simulink model "SMC_simulink_model"  (R2022a)
settings: Solver=VariableStepAuto  StartTime=0.0  StopTime=25  MaxStep=1e-3  RelTol=1e-3
InitFcn:
  | clear
  | clc
  | %% dati
  | w0 = 5.278;
  | alfa1 = w0^2;
  | alfa3 = -1.402*w0^2;
  | alfa5 = 0.271*w0^2;
  | mu1 = 0.086;
  | mu3 = 0.1080;
  | %% parametri SMC
  | mu = 1;
  | P = [1 3]';
  | x0 = [-1.2 -0.18]';
  | xd = [0 0]';
  | %disturbi e variazione parametrica
  | Ad = 0; %ampiezza disturbo
  | fd = 2; %fequenza disturbo
  | epsilon = 0.01; %boundary layer
  | alfa1_hat = 0.8*w0^2
settings Model: Creator=user  LastModifiedBy=user
settings SolverCC: ZeroCrossAlgorithm=Adaptive
settings DebuggingCC: IgnoredZcDiagnostic=none

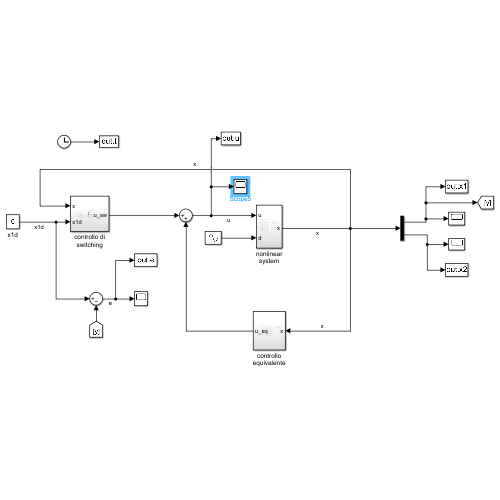
[thumbnail: Simulink's stored preview of the top-level diagram]
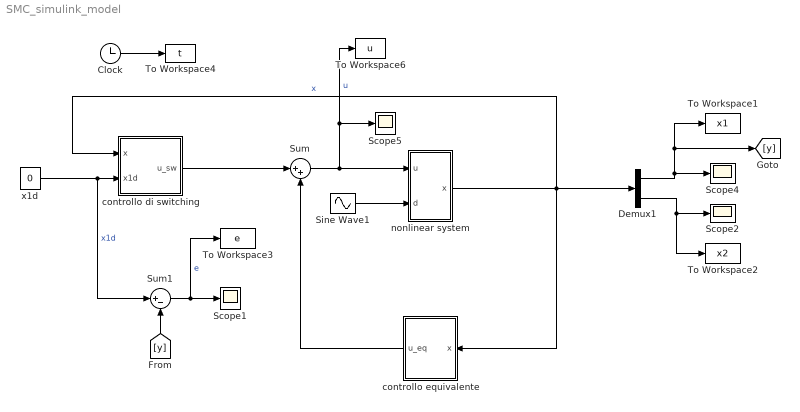
== system SMC_simulink_model ==
  Clock : Clock
  Demux1 : Demux  Outputs=2
  Scope{1..2,4..5} (4 alike) : Scope
  Sine Wave1 : Sin  Amplitude=Ad  Frequency=2  SampleTime=0
  Sum : Sum  Inputs=|++
  Sum1 : Sum  Inputs=|+-
  To Workspace1 : ToWorkspace  VariableName=x1  SampleTime=-1
      settings: Save2DSignal=2-D array (concatenate along first dimension)
  To Workspace2 : ToWorkspace  VariableName=x2  SampleTime=-1
      settings: Save2DSignal=2-D array (concatenate along first dimension)
  To Workspace3 : ToWorkspace  VariableName=e  SampleTime=-1
      settings: Save2DSignal=2-D array (concatenate along first dimension)
  To Workspace4 : ToWorkspace  VariableName=t  SampleTime=-1
      settings: Save2DSignal=2-D array (concatenate along first dimension)
  To Workspace6 : ToWorkspace  VariableName=u  SampleTime=-1
      settings: Save2DSignal=2-D array (concatenate along first dimension)
  controllo equivalente : Subsystem
  controllo di switching : Subsystem
  nonlinear system : Subsystem
  x1d : Constant  Value=0
  wires:
  Demux1/2 -> Scope2/1, To Workspace2/1
  Demux1/1 -> [y], To Workspace1/1, Scope4/1
  x1d/1 -> Sum1/1, controllo di switching/2(x1d)  "x1d"
  nonlinear system/1(x) -> controllo di switching/1(x), Demux1/1, controllo equivalente/1(x)  "x"
  Sum/1 -> To Workspace6/1, Scope5/1, nonlinear system/1(u)  "u"
  controllo di switching/1(u_sw) -> Sum/1
  controllo equivalente/1(u_eq) -> Sum/2
  Sine Wave1/1 -> nonlinear system/2(d)
  Clock/1 -> To Workspace4/1
  Sum1/1 -> To Workspace3/1, Scope1/1  "e"
  [y] -> Sum1/2

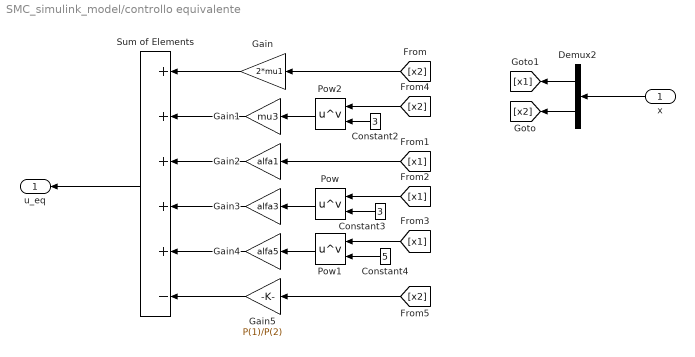
== system SMC_simulink_model/controllo equivalente ==
  x : Inport
  Constant2 : Constant  Value=3
  Constant3 : Constant  Value=3
  Constant4 : Constant  Value=5
  Demux2 : Demux  Outputs=2
  Gain : Gain  Gain=2*mu1
  Gain1 : Gain  Gain=mu3
  Gain2 : Gain  Gain=alfa1
  Gain3 : Gain  Gain=alfa3
  Gain4 : Gain  Gain=alfa5
  Gain5 : Gain  Gain=P(1)/P(2)
  Pow : Math  Operator=pow  RndMeth=Zero
  Pow1 : Math  Operator=pow  RndMeth=Zero
  Pow2 : Math  Operator=pow  RndMeth=Zero
  Sum of Elements : Sum  Inputs=+++++-
  u_eq : Outport
  wires:
  Gain1/1 -> Sum of Elements/2
  [x2] -> Gain/1
  Pow1/1 -> Gain4/1
  Constant2/1 -> Pow2/2
  [x1] -> Gain2/1
  Pow2/1 -> Gain1/1
  [x1] -> Pow/1
  Constant4/1 -> Pow1/2
  Gain5/1 -> Sum of Elements/6
  Constant3/1 -> Pow/2
  Demux2/2 -> [x2]
  Gain4/1 -> Sum of Elements/5
  [x2] -> Gain5/1
  [x1] -> Pow1/1
  Gain/1 -> Sum of Elements/1
  Gain2/1 -> Sum of Elements/3
  Pow/1 -> Gain3/1
  [x2] -> Pow2/1
  Gain3/1 -> Sum of Elements/4
  x/1 -> Demux2/1
  Demux2/1 -> [x1]
  Sum of Elements/1 -> u_eq/1

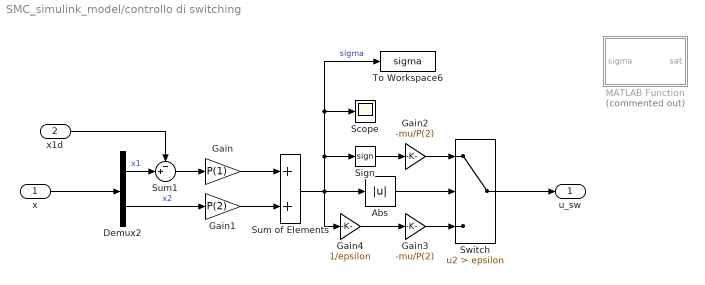
== system SMC_simulink_model/controllo di switching ==
  x : Inport
  x1d : Inport  Port=2
  Abs : Abs  SaturateOnIntegerOverflow=off
  Demux2 : Demux  Outputs=2
  Gain : Gain  Gain=P(1)
  Gain1 : Gain  Gain=P(2)
  Gain2 : Gain  Gain=-mu/P(2)
  Gain3 : Gain  Gain=-mu/P(2)
  Gain4 : Gain  Gain=1/epsilon
  MATLAB Function : MATLAB Function  Commented=on  TreatAsAtomicUnit=on
  Scope : Scope
  Sign : Signum
  Sum of Elements : Sum
  Sum1 : Sum  Inputs=-+|
  Switch : Switch  Criteria=u2 > Threshold  Threshold=epsilon  SaturateOnIntegerOverflow=off  InputSameDT=off
  To Workspace6 : ToWorkspace  VariableName=sigma  SampleTime=-1
      settings: Save2DSignal=2-D array (concatenate along first dimension)
  u_sw : Outport
  wires:
  Sum of Elements/1 -> Gain4/1, Abs/1, Sign/1, To Workspace6/1, Scope/1  "sigma"
  Gain/1 -> Sum of Elements/1
  Demux2/1 -> Sum1/2  "x1"
  Demux2/2 -> Gain1/1  "x2"
  Gain1/1 -> Sum of Elements/2
  Sum1/1 -> Gain/1
  x/1 -> Demux2/1
  x1d/1 -> Sum1/1
  Switch/1 -> u_sw/1
  Gain4/1 -> Gain3/1
  Abs/1 -> Switch/2
  Gain3/1 -> Switch/3
  Gain2/1 -> Switch/1
  Sign/1 -> Gain2/1

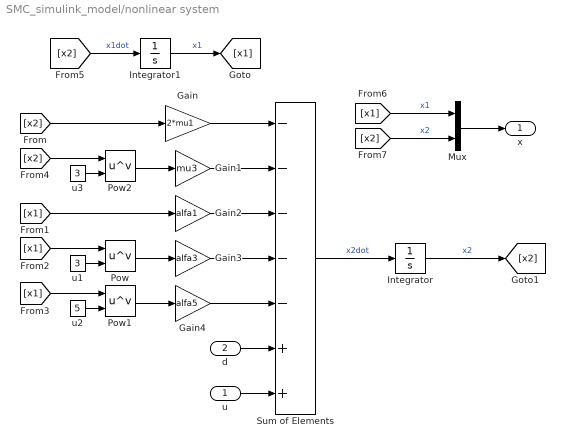
== system SMC_simulink_model/nonlinear system ==
  u : Inport
  d : Inport  Port=2
  Gain : Gain  Gain=2*mu1
  Gain1 : Gain  Gain=mu3
  Gain2 : Gain  Gain=alfa1
  Gain3 : Gain  Gain=alfa3
  Gain4 : Gain  Gain=alfa5
  Integrator : Integrator  InitialCondition=-0.18
  Integrator1 : Integrator  InitialCondition=-1.2
  Mux : Mux  Inputs=2
  Pow : Math  Operator=pow  RndMeth=Zero
  Pow1 : Math  Operator=pow  RndMeth=Zero
  Pow2 : Math  Operator=pow  RndMeth=Zero
  Sum of Elements : Sum  Inputs=-----++
  u1 : Constant  Value=3
  u2 : Constant  Value=5
  u3 : Constant  Value=3
  x : Outport
  wires:
  Gain1/1 -> Sum of Elements/2
  [x2] -> Pow2/1
  u3/1 -> Pow2/2
  [x1] -> Mux/1  "x1"
  [x2] -> Mux/2  "x2"
  Gain/1 -> Sum of Elements/1
  Integrator1/1 -> [x1]  "x1"
  Gain3/1 -> Sum of Elements/4
  Integrator/1 -> [x2]  "x2"
  Pow/1 -> Gain3/1
  u1/1 -> Pow/2
  [x2] -> Integrator1/1  "x1dot"
  Mux/1 -> x/1
  [x1] -> Gain2/1
  [x1] -> Pow1/1
  Sum of Elements/1 -> Integrator/1  "x2dot"
  [x2] -> Gain/1
  Gain2/1 -> Sum of Elements/3
  Pow2/1 -> Gain1/1
  Gain4/1 -> Sum of Elements/5
  Pow1/1 -> Gain4/1
  [x1] -> Pow/1
  u2/1 -> Pow1/2
  u/1 -> Sum of Elements/7
  d/1 -> Sum of Elements/6

== matlab function SMC_simulink_model/controllo di switching/MATLAB Function ==
  data: sigma input; sat output
function sat = fcn(sigma)

mu = 20;
p2 = 3;
epsilon = 0.01;

if sigma > epsilon
    u = -mu/p2;

elseif sigma < -epsilon
    u = mu/p2;

else
    u = -(mu/p2)*(sigma/epsilon);

end

u

sat = u;
